simulink library "PczSimLib_R2020b"  (R2020b)
settings: Solver=VariableStepAuto  StartTime=0.0  StopTime=10.0  RelTol=1e-3
undefined symbols (not defined in the file or in its folder): beta, qc_get_step_size
libraries: dspswit3 x6, pid_lib x4, simulink x3
(part 1 of 2)
settings Model: Creator=SZTAKI  LastModifiedBy=SZTAKI

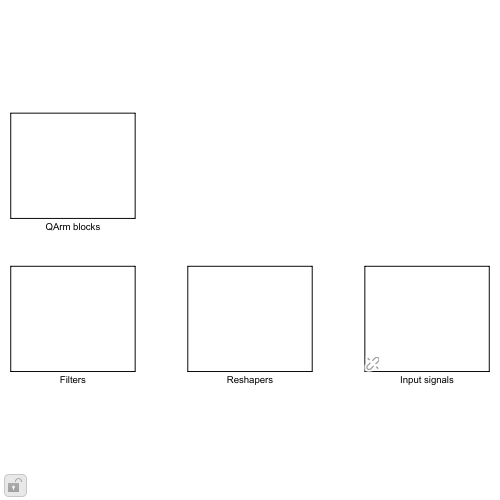
[thumbnail: Simulink's stored preview of the top-level diagram]
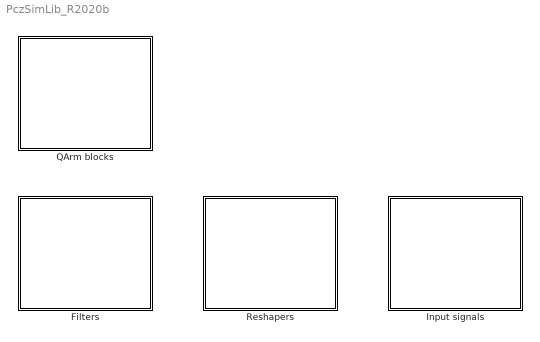
== system PczSimLib_R2020b ==
  Filters : Subsystem
  Input signals : Subsystem  AncestorBlock=PczSimLib_R2020b/Reshapers
  QArm blocks : Subsystem
  Reshapers : Subsystem

== system PczSimLib_R2020b/Filters ==
  Filter Tset = 0.05 [sec] : TransferFcn  Numerator=[0 0 0 1]  Denominator=[5.0000e-07 1.5000e-04 0.0200 1]
  Filter Tset = 0.1 [sec] : TransferFcn  Numerator=[0 0 0 1]  Denominator=[8.5000e-07 2.2000e-04 0.0270 1]
  Filter Tset = 0.25 [sec] : TransferFcn  Numerator=[0 0 0 1]  Denominator=[2.0000e-05 0.0022 0.0800 1]
  Filter Tset = 0.4 [sec] : TransferFcn  Numerator=[0 0 0 1]  Denominator=[7.0000e-05 0.0045 0.1200 1]
  Filter Tset = 0.7 [sec] : TransferFcn  Numerator=[0 0 0 0 0 1]  Denominator=[2.5000e-07 2.5000e-05 0.0011 0.0235 0.2500 1]
  Second-order low-pass filter : Subsystem

== system PczSimLib_R2020b/Input signals ==
  Sigmoid Steps : Subsystem

== system PczSimLib_R2020b/QArm blocks ==
  Current to pwm (corrected) 2022.04.28.1 : Subsystem
  Current transformed to pwm DEPRECATED : Subsystem
  PWM limiter I. : Subsystem
  PWM limiter II. : Subsystem
  Torque to pwm DEPRECATED : Subsystem
  Torque to pwm (J1-3 corrected) DEPRECATED : Subsystem
  Torque to pwm (corrected) 2022.04.28. : Subsystem
  Torque to pwm (corrected) velocity update 2022.05.20. : Subsystem
  "Torque to pwm (corrected) velocity update, current controlled 2022.05.20." : Subsystem
  XM430-W350-R characteristics (wrist) (corrected) : Subsystem
  "XM540-W270-R characteristics (base, shoulder, elbow) (corrected)" : Subsystem
  phi2theta : Subsystem
  theta2phi : Subsystem

== system PczSimLib_R2020b/Reshapers ==
  note: Reshaper = [4 3]; strjoin(cellfun(@(n) {num2str(n)},num2cell(reshape(reshape(1:prod(Reshaper),Reshaper)',[prod(Reshaper) 1])')),',')
  2x4 to 4x2 : Subsystem
  2x8 to 8x2 : Subsystem
  3x4 to 4x3 : Subsystem
  4x4 to 4x4 : Subsystem

== system PczSimLib_R2020b/Filters/Second-order low-pass filter ==
  x : Inport
  wn : Inport  Port=2
  zt : Inport  Port=3
  x0 : Inport  Port=4
  Constant : Constant  Value=2
  Integrator1 : Integrator  InitialConditionSource=external
  Integrator2 : Integrator
  Product : Product  RndMeth=Zero
  Product1 : Product  RndMeth=Zero
  Product2 : Product  Inputs=3  RndMeth=Zero
  Sum : Sum  Inputs=|+-
  Sum1 : Sum  Inputs=|+-
  y : Outport
  yd : Outport  Port=2
  wires:
  x0/1 -> Integrator1/2
  x/1 -> Sum1/1
  Integrator1/1 -> y/1, Sum1/2
  Constant/1 -> Product2/2
  Sum1/1 -> Sum/1
  Product2/1 -> Sum/2
  zt/1 -> Product2/3
  wn/1 -> Product1/1, Product/1
  Product1/1 -> yd/1, Integrator1/1
  Sum/1 -> Product/2
  Integrator2/1 -> Product2/1, Product1/2
  Product/1 -> Integrator2/1

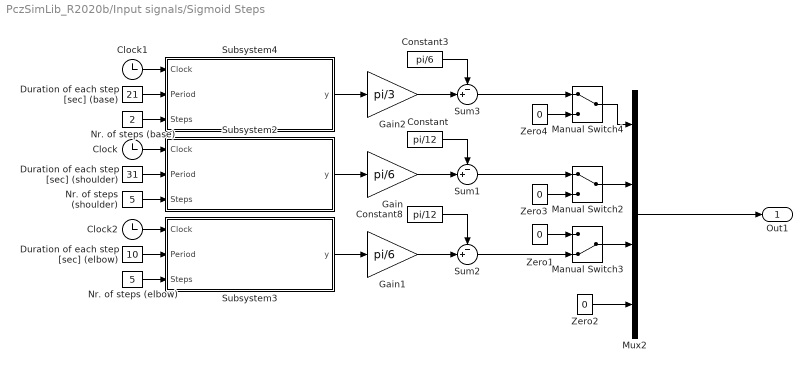
== system PczSimLib_R2020b/Input signals/Sigmoid Steps ==
  Clock : Clock
  Clock1 : Clock
  Clock2 : Clock
  Constant : Constant  Value=pi/12
  Constant3 : Constant  Value=pi/6
  Constant8 : Constant  Value=pi/12
  Duration of each step [sec] (base) : Constant  Value=21
  Duration of each step [sec] (elbow) : Constant  Value=10
  Duration of each step [sec] (shoulder) : Constant  Value=31
  Gain : Gain  Gain=pi/6
  Gain1 : Gain  Gain=pi/6
  Gain2 : Gain  Gain=pi/3
  Manual Switch2 : ManualSwitch
  Manual Switch3 : ManualSwitch  CurrentSetting=0
  Manual Switch4 : ManualSwitch
  Mux2 : Mux
  Nr. of steps (base) : Constant  Value=2
  Nr. of steps (elbow) : Constant  Value=5
  Nr. of steps (shoulder) : Constant  Value=5
  Subsystem2 : Subsystem
  Subsystem3 : Subsystem
  Subsystem4 : Subsystem
  Sum1 : Sum  Inputs=-+|
  Sum2 : Sum  Inputs=-+|
  Sum3 : Sum  Inputs=-+|
  Zero{1..4} (4 alike) : Constant  Value=0  OutDataTypeStr=Inherit: Inherit via back propagation
  Out1 : Outport
  wires:
  Manual Switch2/1 -> Mux2/2
  Duration of each step [sec] (shoulder)/1 -> Subsystem2/2(Period)
  Mux2/1 -> Out1/1
  Nr. of steps (base)/1 -> Subsystem4/3(Steps)
  Constant/1 -> Sum1/1
  Subsystem3/1(y) -> Gain1/1
  Nr. of steps (shoulder)/1 -> Subsystem2/3(Steps)
  Zero4/1 -> Manual Switch4/2
  Sum1/1 -> Manual Switch2/1
  Subsystem2/1(y) -> Gain/1
  Zero1/1 -> Manual Switch3/1
  Clock2/1 -> Subsystem3/1(Clock)
  Clock/1 -> Subsystem2/1(Clock)
  Zero3/1 -> Manual Switch2/2
  Constant3/1 -> Sum3/1
  Clock1/1 -> Subsystem4/1(Clock)
  Gain1/1 -> Sum2/2
  Duration of each step [sec] (elbow)/1 -> Subsystem3/2(Period)
  Subsystem4/1(y) -> Gain2/1
  Sum3/1 -> Manual Switch4/1
  Zero2/1 -> Mux2/4
  Manual Switch4/1 -> Mux2/1
  Constant8/1 -> Sum2/1
  Nr. of steps (elbow)/1 -> Subsystem3/3(Steps)
  Duration of each step [sec] (base)/1 -> Subsystem4/2(Period)
  Gain/1 -> Sum1/2
  Manual Switch3/1 -> Mux2/3
  Gain2/1 -> Sum3/2
  Sum2/1 -> Manual Switch3/2

== system PczSimLib_R2020b/QArm blocks/Current to pwm (corrected) 2022.04.28.1 ==
  current [4] : Inport
  angular vel [4] : Inport  Port=2
  M_curvel2pwm (2022.04.28.) : Constant  Value=|
      | [2.970000e-01,-1.400000e-03, 2.400000e-03,-9.800000e-03
      | -1.000000e-04, 8.800000e-02, 3.500000e-03,-0.000000e+00
      |  7.000000e-04, 8.400000e-03, 1.789000e-01,-2.600000e-03
      |  4.970000e-02, 2.830000e-02, 1.079000e-01, 6.711000e-01
      |  3.084000e-01, 4.800000e-03, 5.600000e-03, 1.100000e-03
      |  8.000000e-04, 3.198000e-01,-4.000000e-04, 5.500000e-03
      | -1.500000e-03,-1.110000e-02, 3.114000e-01, 7.800000e-03
      |  9.000000e-04,-2.300000e-03,-5.100000e-03, 2.074000e-01]'
  Mux2 : Mux  Inputs=2
  Product : Product  Multiplication=Matrix(*)
  pwm [4] : Outport
  wires:
  Mux2/1 -> Product/2
  M_curvel2pwm (2022.04.28.)/1 -> Product/1
  angular vel [4]/1 -> Mux2/2
  current [4]/1 -> Mux2/1
  Product/1 -> pwm [4]/1

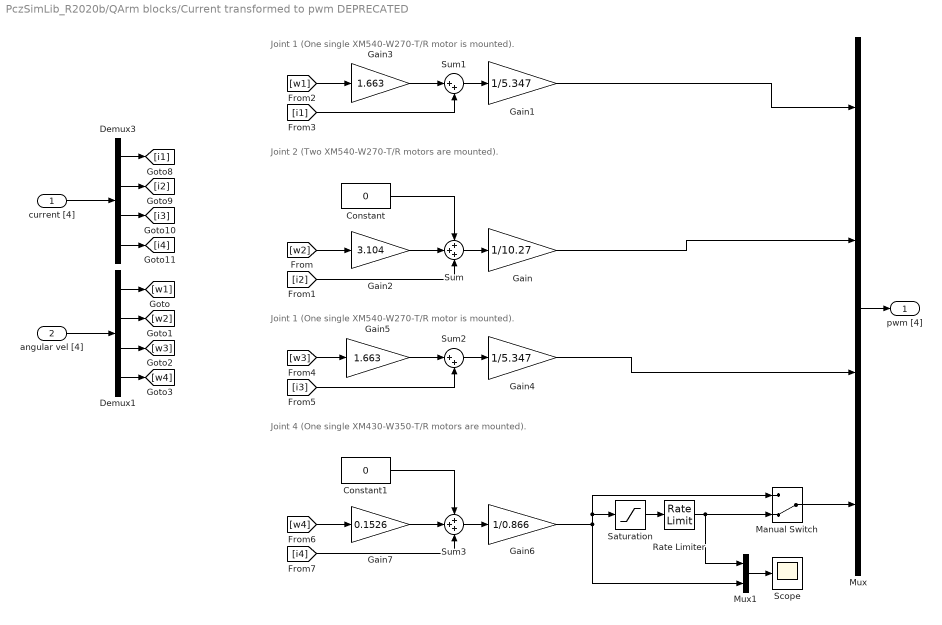
== system PczSimLib_R2020b/QArm blocks/Current transformed to pwm DEPRECATED ==
  note: Joint 4 (One single XM430-W350-T/R motors are mounted).
  note: Joint 1 (One single XM540-W270-T/R motor is mounted).
  note: Joint 1 (One single XM540-W270-T/R motor is mounted).
  note: Joint 2 (Two XM540-W270-T/R motors are mounted).
  current [4] : Inport
  angular vel [4] : Inport  Port=2
  Constant : Constant  Value=0
  Constant1 : Constant  Value=0
  Demux1 : Demux
  Demux3 : Demux
  Gain : Gain  Gain=1/10.27
  Gain1 : Gain  Gain=1/5.347
  Gain2 : Gain  Gain=3.104
  Gain3 : Gain  Gain=1.663
  Gain4 : Gain  Gain=1/5.347
  Gain5 : Gain  Gain=1.663
  Gain6 : Gain  Gain=1/0.866
  Gain7 : Gain  Gain=0.1526
  Manual Switch : ManualSwitch  CurrentSetting=0
  Mux : Mux
  Mux1 : Mux  Inputs=2
  Rate Limiter : RateLimiter  SampleTimeMode=inherited
  Saturation : Saturate  UpperLimit=0.4  LowerLimit=-0.4
  Scope : Scope
  Sum : Sum  Inputs=+++
  Sum1 : Sum  Inputs=|++
  Sum2 : Sum  Inputs=|++
  Sum3 : Sum  Inputs=+++
  pwm [4] : Outport
  wires:
  Manual Switch/1 -> Mux/4
  Mux1/1 -> Scope/1
  Rate Limiter/1 -> Mux1/1, Manual Switch/2
  Saturation/1 -> Rate Limiter/1
  Gain6/1 -> Mux1/2, Saturation/1, Manual Switch/1
  [w4] -> Gain7/1
  Constant1/1 -> Sum3/1
  Gain7/1 -> Sum3/2
  [i4] -> Sum3/3
  Sum3/1 -> Gain6/1
  Mux/1 -> pwm [4]/1
  Gain4/1 -> Mux/3
  Gain/1 -> Mux/2
  Gain1/1 -> Mux/1
  Sum2/1 -> Gain4/1
  [w3] -> Gain5/1
  Gain5/1 -> Sum2/1
  [i3] -> Sum2/2
  [i1] -> Sum1/2
  Gain3/1 -> Sum1/1
  [w1] -> Gain3/1
  Sum1/1 -> Gain1/1
  Sum/1 -> Gain/1
  [i2] -> Sum/3
  Gain2/1 -> Sum/2
  Constant/1 -> Sum/1
  [w2] -> Gain2/1
  current [4]/1 -> Demux3/1
  Demux3/4 -> [i4]
  Demux3/1 -> [i1]
  Demux3/2 -> [i2]
  Demux3/3 -> [i3]
  angular vel [4]/1 -> Demux1/1
  Demux1/1 -> [w1]
  Demux1/2 -> [w2]
  Demux1/3 -> [w3]
  Demux1/4 -> [w4]

== system PczSimLib_R2020b/QArm blocks/PWM limiter I. ==
  pwm in : Inport
  Demux : Demux
  Mux : Mux
  Rate Limiter{,1..3} (4 alike) : RateLimiter  RisingSlewLimit=2  FallingSlewLimit=-2  SampleTimeMode=inherited
  Saturation{,1..3} (4 alike) : Saturate  UpperLimit=0.8  LowerLimit=-0.8
  pwm out : Outport
  wires:
  Demux/4 -> Saturation2/1
  Demux/3 -> Saturation3/1
  Demux/2 -> Saturation1/1
  Demux/1 -> Saturation/1
  pwm in/1 -> Demux/1
  Saturation/1 -> Rate Limiter/1
  Saturation1/1 -> Rate Limiter1/1
  Saturation3/1 -> Rate Limiter2/1
  Saturation2/1 -> Rate Limiter3/1
  Rate Limiter3/1 -> Mux/4
  Rate Limiter2/1 -> Mux/3
  Rate Limiter1/1 -> Mux/2
  Rate Limiter/1 -> Mux/1
  Mux/1 -> pwm out/1

== system PczSimLib_R2020b/QArm blocks/PWM limiter II. ==
  pwm in : Inport
  Demux : Demux
  Mux : Mux
  Rate Limiter : RateLimiter  RisingSlewLimit=2  FallingSlewLimit=-2  SampleTimeMode=inherited
  Rate Limiter1 : RateLimiter  RisingSlewLimit=5  FallingSlewLimit=-5  SampleTimeMode=inherited
  Rate Limiter2 : RateLimiter  RisingSlewLimit=2  FallingSlewLimit=-2  SampleTimeMode=inherited
  Rate Limiter3 : RateLimiter  RisingSlewLimit=2  FallingSlewLimit=-2  SampleTimeMode=inherited
  Saturation{,1..3} (4 alike) : Saturate  UpperLimit=0.8  LowerLimit=-0.8
  pwm out : Outport
  wires:
  Mux/1 -> pwm out/1
  Rate Limiter/1 -> Mux/1
  Rate Limiter1/1 -> Mux/2
  Rate Limiter2/1 -> Mux/3
  Rate Limiter3/1 -> Mux/4
  Saturation2/1 -> Rate Limiter3/1
  Saturation3/1 -> Rate Limiter2/1
  Saturation1/1 -> Rate Limiter1/1
  Saturation/1 -> Rate Limiter/1
  pwm in/1 -> Demux/1
  Demux/1 -> Saturation/1
  Demux/2 -> Saturation1/1
  Demux/3 -> Saturation3/1
  Demux/4 -> Saturation2/1

== system PczSimLib_R2020b/QArm blocks/Torque to pwm DEPRECATED ==
  x [8] : Inport
  u [4] : Inport  Port=2
  params [17] : Inport  Port=3
  Constant1 : Constant  Value=0
  Mux1 : Mux  Inputs=2
  Selector : Selector  InputPortWidth=4  IndexOptions=Index vector (dialog)  Indices=1:3  OutputSizes=1
  Selector1 : Selector  InputPortWidth=8  IndexOptions=Index vector (dialog)  Indices=5:8  OutputSizes=1
  Selector2 : Selector  InputPortWidth=4  IndexOptions=Index vector (dialog)  Indices=4  OutputSizes=1
  Tau(u,x) : MATLAB Function  TreatAsAtomicUnit=on
  XM430-W350-R characteristics (corrected) : Subsystem
  XM540-W270-R characteristics (corrected) : Subsystem
  current transformed to pwm (corrected) : Subsystem
  pwm [4] : Outport
  i [4] : Outport  Port=2
  tau [4] : Outport  Port=3
  wires:
  current transformed to pwm (corrected)/1(pwm [4]) -> pwm [4]/1
  Mux1/1 -> i [4]/1, current transformed to pwm (corrected)/1(current [4])
  x [8]/1 -> Selector1/1, Tau(u,x)/3(x)
  Constant1/1 -> Tau(u,x)/4(mL)
  Selector/1 -> XM540-W270-R characteristics (corrected)/1(torque [3])
  XM540-W270-R characteristics (corrected)/1(current [3]) -> Mux1/1
  u [4]/1 -> Tau(u,x)/2(u)
  Tau(u,x)/1(Tau) -> tau [4]/1, Selector2/1, Selector/1  "Tau"
  Selector1/1 -> current transformed to pwm (corrected)/2(angular vel [4])
  Selector2/1 -> XM430-W350-R characteristics (corrected)/1(wrist torque)
  XM430-W350-R characteristics (corrected)/1(wrist current) -> Mux1/2
  params [17]/1 -> Tau(u,x)/1(params)

== system PczSimLib_R2020b/QArm blocks/Torque to pwm (J1-3 corrected) DEPRECATED ==
  x [8] : Inport
  u [4] : Inport  Port=2
  params [17] : Inport  Port=3
  Constant1 : Constant  Value=0
  Mux1 : Mux  Inputs=2
  Selector : Selector  InputPortWidth=4  IndexOptions=Index vector (dialog)  Indices=1:3  OutputSizes=1
  Selector1 : Selector  InputPortWidth=8  IndexOptions=Index vector (dialog)  Indices=5:8  OutputSizes=1
  Selector2 : Selector  InputPortWidth=4  IndexOptions=Index vector (dialog)  Indices=4  OutputSizes=1
  Tau(u,x) : MATLAB Function  TreatAsAtomicUnit=on
  XM430-W350-R characteristics (corrected) : Subsystem
  XM540-W270-R characteristics (corrected) : Subsystem
  current transformed to pwm (corrected) : Subsystem
  pwm [4] : Outport
  i [4] : Outport  Port=2
  tau [4] : Outport  Port=3
  wires:
  params [17]/1 -> Tau(u,x)/1(params)
  XM430-W350-R characteristics (corrected)/1(wrist current) -> Mux1/2
  Selector2/1 -> XM430-W350-R characteristics (corrected)/1(wrist torque)
  Selector1/1 -> current transformed to pwm (corrected)/2(angular vel [4])
  Tau(u,x)/1(Tau) -> Selector/1, Selector2/1, tau [4]/1  "Tau"
  u [4]/1 -> Tau(u,x)/2(u)
  XM540-W270-R characteristics (corrected)/1(current [3]) -> Mux1/1
  Selector/1 -> XM540-W270-R characteristics (corrected)/1(torque [3])
  Constant1/1 -> Tau(u,x)/4(mL)
  x [8]/1 -> Tau(u,x)/3(x), Selector1/1
  Mux1/1 -> current transformed to pwm (corrected)/1(current [4]), i [4]/1
  current transformed to pwm (corrected)/1(pwm [4]) -> pwm [4]/1

== system PczSimLib_R2020b/QArm blocks/Torque to pwm (corrected) 2022.04.28. ==
  x [8] : Inport
  u [4] : Inport  Port=2
  params [17] : Inport  Port=3
  Constant1 : Constant  Value=0
  Current to pwm (corrected) 2022.04.28. : Subsystem
  Mux1 : Mux  Inputs=2
  Selector : Selector  InputPortWidth=4  IndexOptions=Index vector (dialog)  Indices=1:3  OutputSizes=1
  Selector1 : Selector  InputPortWidth=8  IndexOptions=Index vector (dialog)  Indices=5:8  OutputSizes=1
  Selector2 : Selector  InputPortWidth=4  IndexOptions=Index vector (dialog)  Indices=4  OutputSizes=1
  Tau(u,x) : MATLAB Function  TreatAsAtomicUnit=on
  XM430-W350-R characteristics (corrected) : Subsystem
  XM540-W270-R characteristics (corrected) : Subsystem
  pwm [4] : Outport
  i [4] : Outport  Port=2
  tau [4] : Outport  Port=3
  wires:
  Current to pwm (corrected) 2022.04.28./1(pwm [4]) -> pwm [4]/1
  Mux1/1 -> Current to pwm (corrected) 2022.04.28./1(current [4]), i [4]/1
  x [8]/1 -> Selector1/1, Tau(u,x)/3(x)
  Constant1/1 -> Tau(u,x)/4(mL)
  Selector/1 -> XM540-W270-R characteristics (corrected)/1(torque [3])
  XM540-W270-R characteristics (corrected)/1(current [3]) -> Mux1/1
  u [4]/1 -> Tau(u,x)/2(u)
  Tau(u,x)/1(Tau) -> tau [4]/1, Selector2/1, Selector/1  "Tau"
  Selector1/1 -> Current to pwm (corrected) 2022.04.28./2(angular vel [4])
  Selector2/1 -> XM430-W350-R characteristics (corrected)/1(wrist torque)
  XM430-W350-R characteristics (corrected)/1(wrist current) -> Mux1/2
  params [17]/1 -> Tau(u,x)/1(params)

== system PczSimLib_R2020b/QArm blocks/Torque to pwm (corrected) velocity update 2022.05.20. ==
  x (Tc) [8] : Inport
  u (Tc) [4] : Inport  Port=2
  params [17] : Inport  Port=3
  w (Ts) [4] : Inport  Port=4
  Constant1 : Constant  Value=0
  Current to pwm (corrected) 2022.04.28. : Subsystem
  Mux1 : Mux  Inputs=2
  "Oversampling (Tc -> Ts)" : RateTransition  OutPortSampleTime=qc_get_step_size
  Selector : Selector  InputPortWidth=4  IndexOptions=Index vector (dialog)  Indices=1:3  OutputSizes=1
  Selector2 : Selector  InputPortWidth=4  IndexOptions=Index vector (dialog)  Indices=4  OutputSizes=1
  Tau(u,x) : MATLAB Function  TreatAsAtomicUnit=on
  XM430-W350-R characteristics (corrected) : Subsystem
  XM540-W270-R characteristics (corrected) : Subsystem
  pwm [4] : Outport
  i [4] : Outport  Port=2
  tau [4] : Outport  Port=3
  wires:
  params [17]/1 -> Tau(u,x)/1(params)
  XM430-W350-R characteristics (corrected)/1(wrist current) -> Mux1/2
  Selector2/1 -> XM430-W350-R characteristics (corrected)/1(wrist torque)
  Tau(u,x)/1(Tau) -> Selector/1, Selector2/1, tau [4]/1  "Tau"
  u (Tc) [4]/1 -> Tau(u,x)/2(u)
  XM540-W270-R characteristics (corrected)/1(current [3]) -> Mux1/1
  Selector/1 -> XM540-W270-R characteristics (corrected)/1(torque [3])
  Constant1/1 -> Tau(u,x)/4(mL)
  x (Tc) [8]/1 -> Tau(u,x)/3(x)
  Mux1/1 -> "Oversampling (Tc -> Ts)"/1, i [4]/1
  Current to pwm (corrected) 2022.04.28./1(pwm [4]) -> pwm [4]/1
  "Oversampling (Tc -> Ts)"/1 -> Current to pwm (corrected) 2022.04.28./1(current [4])
  w (Ts) [4]/1 -> Current to pwm (corrected) 2022.04.28./2(angular vel [4])

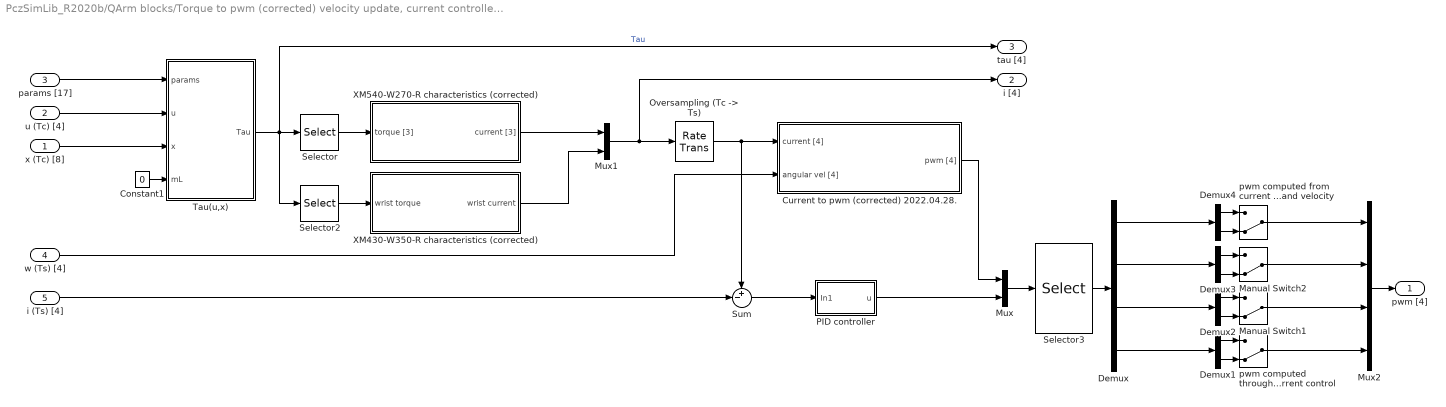
== system PczSimLib_R2020b/QArm blocks/Torque to pwm (corrected) velocity update, current controlled 2022.05.20. ==
  x (Tc) [8] : Inport
  u (Tc) [4] : Inport  Port=2
  params [17] : Inport  Port=3
  w (Ts) [4] : Inport  Port=4
  i (Ts) [4] : Inport  Port=5
  Constant1 : Constant  Value=0
  Current to pwm (corrected) 2022.04.28. : Subsystem
  Demux : Demux  Outputs=[2 2 2 2]
  Demux{1..4} (4 alike) : Demux  Outputs=2
  Manual Switch1 : ManualSwitch  CurrentSetting=0
  Manual Switch2 : ManualSwitch  CurrentSetting=0
  Mux : Mux  Inputs=2
  Mux1 : Mux  Inputs=2
  Mux2 : Mux
  "Oversampling (Tc -> Ts)" : RateTransition  OutPortSampleTime=qc_get_step_size
  PID controller : Subsystem
  Selector : Selector  InputPortWidth=4  IndexOptions=Index vector (dialog)  Indices=1:3  OutputSizes=1
  Selector2 : Selector  InputPortWidth=4  IndexOptions=Index vector (dialog)  Indices=4  OutputSizes=1
  Selector3 : Selector  InputPortWidth=8  IndexOptions=Index vector (dialog)  Indices=[1,5,2,6,3,7,4,8]  OutputSizes=1
  Sum : Sum  Inputs=+-|
  Tau(u,x) : MATLAB Function  TreatAsAtomicUnit=on
  XM430-W350-R characteristics (corrected) : Subsystem
  XM540-W270-R characteristics (corrected) : Subsystem
  pwm computed from current and velocity : ManualSwitch  CurrentSetting=0
  pwm computed through PID-based current control : ManualSwitch  CurrentSetting=0
  pwm [4] : Outport
  i [4] : Outport  Port=2
  tau [4] : Outport  Port=3
  wires:
  w (Ts) [4]/1 -> Current to pwm (corrected) 2022.04.28./2(angular vel [4])
  "Oversampling (Tc -> Ts)"/1 -> Current to pwm (corrected) 2022.04.28./1(current [4]), Sum/1
  Mux1/1 -> i [4]/1, "Oversampling (Tc -> Ts)"/1
  x (Tc) [8]/1 -> Tau(u,x)/3(x)
  Constant1/1 -> Tau(u,x)/4(mL)
  Selector/1 -> XM540-W270-R characteristics (corrected)/1(torque [3])
  XM540-W270-R characteristics (corrected)/1(current [3]) -> Mux1/1
  u (Tc) [4]/1 -> Tau(u,x)/2(u)
  Tau(u,x)/1(Tau) -> tau [4]/1, Selector2/1, Selector/1  "Tau"
  Selector2/1 -> XM430-W350-R characteristics (corrected)/1(wrist torque)
  XM430-W350-R characteristics (corrected)/1(wrist current) -> Mux1/2
  params [17]/1 -> Tau(u,x)/1(params)
  Manual Switch1/1 -> Mux2/3
  Manual Switch2/1 -> Mux2/2
  pwm computed through PID-based current control/1 -> Mux2/4
  Demux/4 -> Demux1/1
  Demux1/2 -> pwm computed through PID-based current control/2
  Demux/2 -> Demux3/1
  Current to pwm (corrected) 2022.04.28./1(pwm [4]) -> Mux/1
  PID controller/1(u) -> Mux/2
  Demux2/1 -> Manual Switch1/1
  Demux3/2 -> Manual Switch2/2
  Demux1/1 -> pwm computed through PID-based current control/1
  Demux3/1 -> Manual Switch2/1
  Demux2/2 -> Manual Switch1/2
  Demux/3 -> Demux2/1
  Selector3/1 -> Demux/1
  Mux/1 -> Selector3/1
  Demux/1 -> Demux4/1
  Demux4/1 -> pwm computed from current and velocity/1
  Demux4/2 -> pwm computed from current and velocity/2
  pwm computed from current and velocity/1 -> Mux2/1
  Mux2/1 -> pwm [4]/1
  Sum/1 -> PID controller/1(In1)
  i (Ts) [4]/1 -> Sum/2

== system PczSimLib_R2020b/QArm blocks/XM430-W350-R characteristics (wrist) (corrected) ==
  wrist torque : Inport
  Abs : Abs
  Constant : Constant  Value=0.0799
  Gain : Gain  Gain=1.7143
  Gain2 : Gain  Gain=0.5734
  Product : Product
  Sign : Signum
  Sum1 : Sum  Inputs=++|
  Switch : Switch  Criteria=u2 > Threshold  Threshold=0.07
  wrist current : Outport
  wires:
  Sign/1 -> Product/2
  Abs/1 -> Gain2/1, Gain/1, Switch/2
  Product/1 -> wrist current/1
  Constant/1 -> Sum1/1
  Gain2/1 -> Sum1/2
  wrist torque/1 -> Sign/1, Abs/1
  Gain/1 -> Switch/3
  Switch/1 -> Product/1  "wrist current"
  Sum1/1 -> Switch/1

== system PczSimLib_R2020b/QArm blocks/XM540-W270-R characteristics (base, shoulder, elbow) (corrected) ==
  torque [3] : Inport
  Abs : Abs
  Constant : Constant  Value=0.1461
  Gain : Gain  Gain=0.6788
  Gain1 : Gain  Gain=0.01717
  Gain2 : Gain  Gain=0.3067
  Product : Product
  Sign : Signum
  Square : Math  Operator=square  SaturateOnIntegerOverflow=on
  Sum1 : Sum  Inputs=+++
  Switch : Switch  Criteria=u2 > Threshold  Threshold=0.4
  current [3] : Outport
  wires:
  Product/1 -> current [3]/1
  Sign/1 -> Product/2
  torque [3]/1 -> Abs/1, Sign/1
  Sum1/1 -> Switch/1
  Switch/1 -> Product/1  "current [3]"
  Square/1 -> Gain1/1
  Gain/1 -> Switch/3
  Gain2/1 -> Sum1/3
  Gain1/1 -> Sum1/2
  Abs/1 -> Switch/2, Gain2/1, Square/1, Gain/1
  Constant/1 -> Sum1/1

== system PczSimLib_R2020b/QArm blocks/phi2theta ==
  phi : Inport
  Constant5 : Constant  Value=beta
  Constant6 : Constant  Value=pi/2
  Demux : Demux
  Mux3 : Mux
  Sum : Sum  Inputs=-++
  Sum1 : Sum  Inputs=-+|
  theta : Outport
  wires:
  Sum/1 -> Mux3/2  "theta2"
  Sum1/1 -> Mux3/3  "theta3"
  Demux/3 -> Sum1/2  "phi3"
  Constant5/1 -> Sum/3, Sum1/1
  Constant6/1 -> Sum/1
  Demux/2 -> Sum/2  "phi2"
  Demux/1 -> Mux3/1  "phi1 = theta1"
  Demux/4 -> Mux3/4  "phi4 = theta4"
  Mux3/1 -> theta/1
  phi/1 -> Demux/1

== system PczSimLib_R2020b/QArm blocks/theta2phi ==
  theta : Inport
  Constant5 : Constant  Value=beta
  Constant6 : Constant  Value=pi/2
  Demux : Demux
  Mux3 : Mux
  Sum : Sum  Inputs=++-
  Sum1 : Sum  Inputs=++|
  phi : Outport
  wires:
  theta/1 -> Demux/1
  Mux3/1 -> phi/1
  Demux/4 -> Mux3/4  "theta4 = phi4"
  Demux/1 -> Mux3/1  "theta1 = phi1"
  Demux/2 -> Sum/2  "theta2"
  Constant6/1 -> Sum/1
  Constant5/1 -> Sum1/1, Sum/3
  Demux/3 -> Sum1/2  "theta3"
  Sum1/1 -> Mux3/3  "phi3"
  Sum/1 -> Mux3/2  "phi2"

== system PczSimLib_R2020b/Reshapers/2x4 to 4x2 ==
  Input 1 [4] : Inport
  Input 2 [4] : Inport  Port=2
  Demux : Demux  Outputs=[2 2 2 2]
  Mux : Mux  Inputs=2
  Reshape block vector (2x4 to 4x2) : Selector  InputPortWidth=8  IndexOptions=Index vector (dialog)  Indices=[1,5,2,6,3,7,4,8]  OutputSizes=1
  Out1 : Outport
  Out2 : Outport  Port=2
  Out3 : Outport  Port=3
  Out4 : Outport  Port=4
  wires:
  Demux/4 -> Out4/1
  Demux/3 -> Out3/1
  Demux/2 -> Out2/1
  Demux/1 -> Out1/1
  Reshape block vector (2x4 to 4x2)/1 -> Demux/1
  Mux/1 -> Reshape block vector (2x4 to 4x2)/1
  Input 2 [4]/1 -> Mux/2
  Input 1 [4]/1 -> Mux/1

== system PczSimLib_R2020b/Reshapers/2x8 to 8x2 ==
  Input 1 [8] : Inport
  Input 2 [8] : Inport  Port=2
  Demux : Demux  Outputs=[2 2 2 2 2 2 2 2]
  Mux : Mux  Inputs=2
  Reshape block vector (2x8 to 8x2) : Selector  InputPortWidth=16  IndexOptions=Index vector (dialog)  Indices=[1,9,2,10,3,11,4,12,5,13,6,14,7,15,8,16]  OutputSizes=1
  Out1 : Outport
  Out2 : Outport  Port=2
  Out3 : Outport  Port=3
  Out4 : Outport  Port=4
  Out5 : Outport  Port=5
  Out6 : Outport  Port=6
  Out7 : Outport  Port=7
  Out8 : Outport  Port=8
  wires:
  Input 1 [8]/1 -> Mux/1
  Input 2 [8]/1 -> Mux/2
  Mux/1 -> Reshape block vector (2x8 to 8x2)/1
  Reshape block vector (2x8 to 8x2)/1 -> Demux/1
  Demux/1 -> Out1/1
  Demux/2 -> Out2/1
  Demux/3 -> Out3/1
  Demux/4 -> Out4/1
  Demux/5 -> Out5/1
  Demux/6 -> Out6/1
  Demux/7 -> Out7/1
  Demux/8 -> Out8/1

== system PczSimLib_R2020b/Reshapers/3x4 to 4x3 ==
  Input 1 [4] : Inport
  Input 2 [4] : Inport  Port=2
  Input 3 [4] : Inport  Port=3
  Demux : Demux  Outputs=[3 3 3 3]
  Mux : Mux  Inputs=3
  Transpose block vector (3x4 to 4x3) : Selector  InputPortWidth=12  IndexOptions=Index vector (dialog)  Indices=[1,5,9,2,6,10,3,7,11,4,8,12]  OutputSizes=1
  Out1 : Outport
  Out2 : Outport  Port=2
  Out3 : Outport  Port=3
  Out4 : Outport  Port=4
  wires:
  Input 1 [4]/1 -> Mux/1
  Input 2 [4]/1 -> Mux/2
  Mux/1 -> Transpose block vector (3x4 to 4x3)/1
  Transpose block vector (3x4 to 4x3)/1 -> Demux/1
  Demux/1 -> Out1/1
  Demux/2 -> Out2/1
  Demux/3 -> Out3/1
  Demux/4 -> Out4/1
  Input 3 [4]/1 -> Mux/3

== system PczSimLib_R2020b/Reshapers/4x4 to 4x4 ==
  Input 1 [4] : Inport
  Input 2 [4] : Inport  Port=2
  Input 3 [4] : Inport  Port=3
  Input 4 [4] : Inport  Port=4
  Demux : Demux  Outputs=[4 4 4 4]
  Mux : Mux
  Transpose block vector (4x4 to 4x4) : Selector  InputPortWidth=16  IndexOptions=Index vector (dialog)  Indices=[1,5,9,13,2,6,10,14,3,7,11,15,4,8,12,16]  OutputSizes=1
  Out1 : Outport
  Out2 : Outport  Port=2
  Out3 : Outport  Port=3
  Out4 : Outport  Port=4
  wires:
  Input 4 [4]/1 -> Mux/4
  Input 3 [4]/1 -> Mux/3
  Demux/4 -> Out4/1
  Demux/3 -> Out3/1
  Demux/2 -> Out2/1
  Demux/1 -> Out1/1
  Transpose block vector (4x4 to 4x4)/1 -> Demux/1
  Mux/1 -> Transpose block vector (4x4 to 4x4)/1
  Input 2 [4]/1 -> Mux/2
  Input 1 [4]/1 -> Mux/1

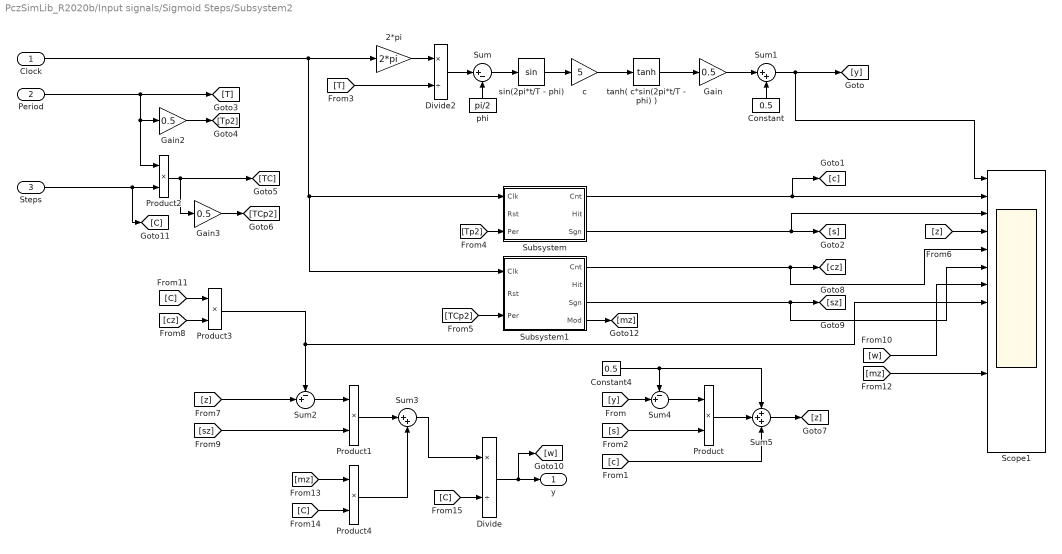
== system PczSimLib_R2020b/Input signals/Sigmoid Steps/Subsystem2 ==
  Clock : Inport
  Period : Inport  Port=2
  Steps : Inport  Port=3
  2*pi : Gain  Gain=2*pi
  Constant : Constant  Value=0.5
  Constant4 : Constant  Value=0.5
  Divide : Product  Inputs=*/
  Divide2 : Product  Inputs=*/
  Gain : Gain  Gain=0.5
  Gain2 : Gain  Gain=0.5
  Gain3 : Gain  Gain=0.5
  Product{,1..4} (5 alike) : Product
  Scope1 : Scope  NumInputPorts=16
  Subsystem : Subsystem
  Subsystem1 : Subsystem
  Sum : Sum  Inputs=|+-
  Sum1 : Sum  Inputs=|++
  Sum2 : Sum  Inputs=-+|
  Sum3 : Sum  Inputs=|++
  Sum4 : Sum  Inputs=-+|
  Sum5 : Sum  Inputs=+++
  c : Gain  Gain=5
  phi : Constant  Value=pi/2  OutDataTypeStr=Inherit: Inherit via back propagation
  sin(2pi*t/T - phi) : Trigonometry
  tanh( c*sin(2pi*t/T - phi) ) : Trigonometry  Operator=tanh
  y : Outport
  wires:
  [mz] -> Scope1/12
  Sum5/1 -> [z]
  [y] -> Sum4/2
  [C] -> Product3/1
  c/1 -> tanh( c*sin(2pi*t/T - phi) )/1
  Constant/1 -> Sum1/2
  Sum3/1 -> Divide/1
  [cz] -> Product3/2
  [z] -> Sum2/2
  Subsystem/3(Sgn) -> Scope1/3, [s]
  [s] -> Product/2
  Product1/1 -> Sum3/1
  Clock/1 -> Subsystem1/1(Clk), Subsystem/1(Clk), 2*pi/1
  Subsystem1/3(Sgn) -> Scope1/6, [sz]
  Sum2/1 -> Product1/1
  Product3/1 -> Sum2/1, Scope1/8
  Constant4/1 -> Sum5/1, Sum4/1
  Gain3/1 -> [TCp2]
  [z] -> Scope1/4
  sin(2pi*t/T - phi)/1 -> c/1
  2*pi/1 -> Divide2/1
  [T] -> Divide2/2
  [sz] -> Product1/2
  [c] -> Sum5/3
  [TCp2] -> Subsystem1/3(Per)
  Period/1 -> Product2/1, Gain2/1, [T]
  [mz] -> Product4/1
  Product4/1 -> Sum3/2
  Gain/1 -> Sum1/1
  phi/1 -> Sum/2
  Product/1 -> Sum5/2
  Subsystem1/1(Cnt) -> Scope1/5, [cz]
  Divide2/1 -> Sum/1
  [C] -> Product4/2
  tanh( c*sin(2pi*t/T - phi) )/1 -> Gain/1
  [Tp2] -> Subsystem/3(Per)
  Sum/1 -> sin(2pi*t/T - phi)/1
  Sum1/1 -> Scope1/1, [y]
  Gain2/1 -> [Tp2]
  Sum4/1 -> Product/1
  Steps/1 -> [C], Product2/2
  Subsystem1/4(Mod) -> [mz]
  [w] -> Scope1/7
  Product2/1 -> Gain3/1, [TC]
  Subsystem/1(Cnt) -> [c], Scope1/2
  Divide/1 -> y/1, [w]
  [C] -> Divide/2

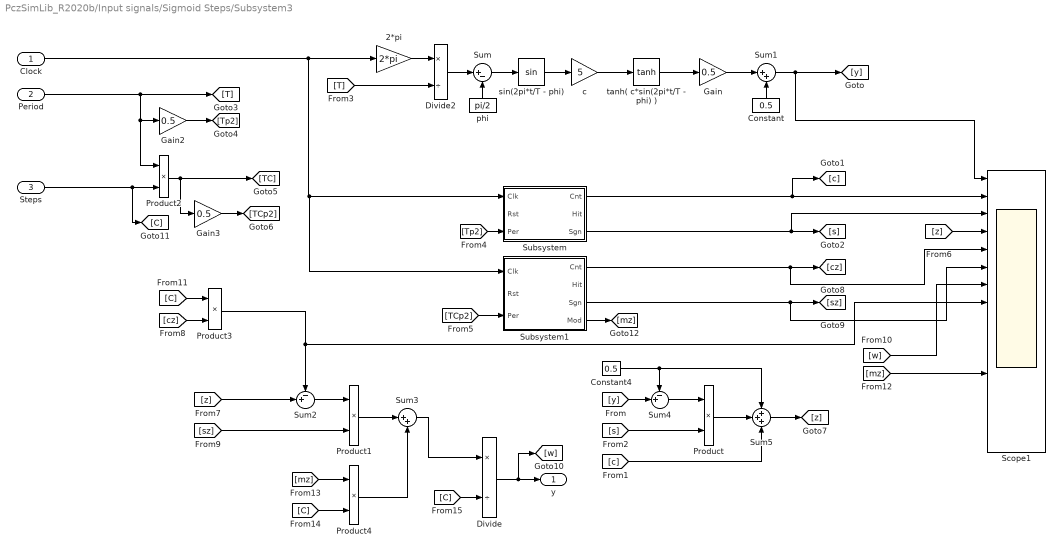
== system PczSimLib_R2020b/Input signals/Sigmoid Steps/Subsystem3 ==
  Clock : Inport
  Period : Inport  Port=2
  Steps : Inport  Port=3
  2*pi : Gain  Gain=2*pi
  Constant : Constant  Value=0.5
  Constant4 : Constant  Value=0.5
  Divide : Product  Inputs=*/
  Divide2 : Product  Inputs=*/
  Gain : Gain  Gain=0.5
  Gain2 : Gain  Gain=0.5
  Gain3 : Gain  Gain=0.5
  Product{,1..4} (5 alike) : Product
  Scope1 : Scope  NumInputPorts=16
  Subsystem : Subsystem
  Subsystem1 : Subsystem
  Sum : Sum  Inputs=|+-
  Sum1 : Sum  Inputs=|++
  Sum2 : Sum  Inputs=-+|
  Sum3 : Sum  Inputs=|++
  Sum4 : Sum  Inputs=-+|
  Sum5 : Sum  Inputs=+++
  c : Gain  Gain=5
  phi : Constant  Value=pi/2  OutDataTypeStr=Inherit: Inherit via back propagation
  sin(2pi*t/T - phi) : Trigonometry
  tanh( c*sin(2pi*t/T - phi) ) : Trigonometry  Operator=tanh
  y : Outport
  wires:
  [C] -> Divide/2
  Divide/1 -> [w], y/1
  Subsystem/1(Cnt) -> Scope1/2, [c]
  Product2/1 -> [TC], Gain3/1
  [w] -> Scope1/7
  Subsystem1/4(Mod) -> [mz]
  Steps/1 -> Product2/2, [C]
  Sum4/1 -> Product/1
  Gain2/1 -> [Tp2]
  Sum1/1 -> [y], Scope1/1
  Sum/1 -> sin(2pi*t/T - phi)/1
  [Tp2] -> Subsystem/3(Per)
  tanh( c*sin(2pi*t/T - phi) )/1 -> Gain/1
  [C] -> Product4/2
  Divide2/1 -> Sum/1
  Subsystem1/1(Cnt) -> [cz], Scope1/5
  Product/1 -> Sum5/2
  phi/1 -> Sum/2
  Gain/1 -> Sum1/1
  Product4/1 -> Sum3/2
  [mz] -> Product4/1
  Period/1 -> [T], Gain2/1, Product2/1
  [TCp2] -> Subsystem1/3(Per)
  [c] -> Sum5/3
  [sz] -> Product1/2
  [T] -> Divide2/2
  2*pi/1 -> Divide2/1
  sin(2pi*t/T - phi)/1 -> c/1
  [z] -> Scope1/4
  Gain3/1 -> [TCp2]
  Constant4/1 -> Sum4/1, Sum5/1
  Product3/1 -> Scope1/8, Sum2/1
  Sum2/1 -> Product1/1
  Subsystem1/3(Sgn) -> [sz], Scope1/6
  Clock/1 -> 2*pi/1, Subsystem/1(Clk), Subsystem1/1(Clk)
  Product1/1 -> Sum3/1
  [s] -> Product/2
  Subsystem/3(Sgn) -> [s], Scope1/3
  [z] -> Sum2/2
  [cz] -> Product3/2
  Sum3/1 -> Divide/1
  Constant/1 -> Sum1/2
  c/1 -> tanh( c*sin(2pi*t/T - phi) )/1
  [C] -> Product3/1
  [y] -> Sum4/2
  Sum5/1 -> [z]
  [mz] -> Scope1/12

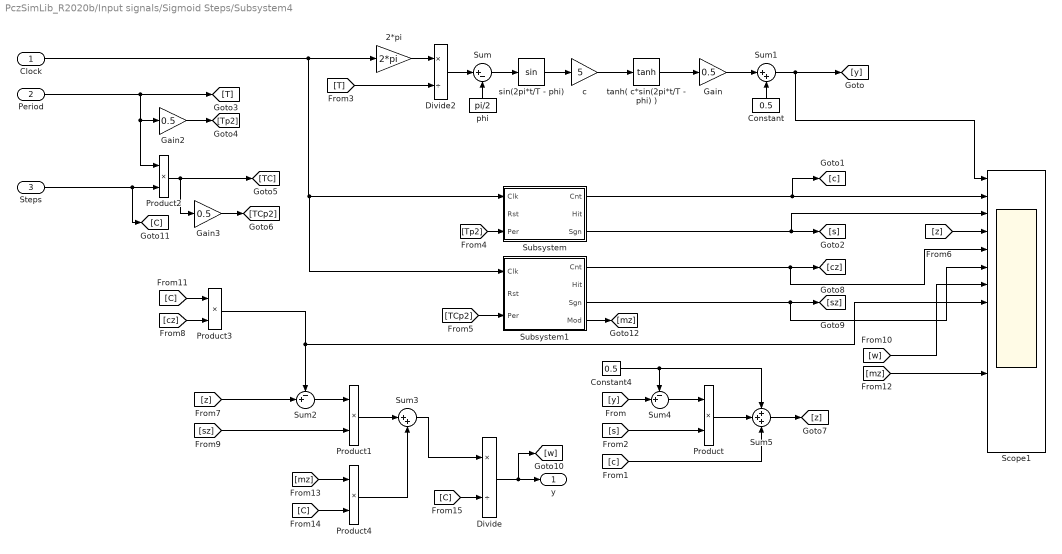
== system PczSimLib_R2020b/Input signals/Sigmoid Steps/Subsystem4 ==
  Clock : Inport
  Period : Inport  Port=2
  Steps : Inport  Port=3
  2*pi : Gain  Gain=2*pi
  Constant : Constant  Value=0.5
  Constant4 : Constant  Value=0.5
  Divide : Product  Inputs=*/
  Divide2 : Product  Inputs=*/
  Gain : Gain  Gain=0.5
  Gain2 : Gain  Gain=0.5
  Gain3 : Gain  Gain=0.5
  Product{,1..4} (5 alike) : Product
  Scope1 : Scope  NumInputPorts=16
  Subsystem : Subsystem
  Subsystem1 : Subsystem
  Sum : Sum  Inputs=|+-
  Sum1 : Sum  Inputs=|++
  Sum2 : Sum  Inputs=-+|
  Sum3 : Sum  Inputs=|++
  Sum4 : Sum  Inputs=-+|
  Sum5 : Sum  Inputs=+++
  c : Gain  Gain=5
  phi : Constant  Value=pi/2  OutDataTypeStr=Inherit: Inherit via back propagation
  sin(2pi*t/T - phi) : Trigonometry
  tanh( c*sin(2pi*t/T - phi) ) : Trigonometry  Operator=tanh
  y : Outport
  wires:
  [C] -> Divide/2
  Divide/1 -> [w], y/1
  Subsystem/1(Cnt) -> Scope1/2, [c]
  Product2/1 -> [TC], Gain3/1
  [w] -> Scope1/7
  Subsystem1/4(Mod) -> [mz]
  Steps/1 -> Product2/2, [C]
  Sum4/1 -> Product/1
  Gain2/1 -> [Tp2]
  Sum1/1 -> [y], Scope1/1
  Sum/1 -> sin(2pi*t/T - phi)/1
  [Tp2] -> Subsystem/3(Per)
  tanh( c*sin(2pi*t/T - phi) )/1 -> Gain/1
  [C] -> Product4/2
  Divide2/1 -> Sum/1
  Subsystem1/1(Cnt) -> [cz], Scope1/5
  Product/1 -> Sum5/2
  phi/1 -> Sum/2
  Gain/1 -> Sum1/1
  Product4/1 -> Sum3/2
  [mz] -> Product4/1
  Period/1 -> [T], Gain2/1, Product2/1
  [TCp2] -> Subsystem1/3(Per)
  [c] -> Sum5/3
  [sz] -> Product1/2
  [T] -> Divide2/2
  2*pi/1 -> Divide2/1
  sin(2pi*t/T - phi)/1 -> c/1
  [z] -> Scope1/4
  Gain3/1 -> [TCp2]
  Constant4/1 -> Sum4/1, Sum5/1
  Product3/1 -> Scope1/8, Sum2/1
  Sum2/1 -> Product1/1
  Subsystem1/3(Sgn) -> [sz], Scope1/6
  Clock/1 -> 2*pi/1, Subsystem/1(Clk), Subsystem1/1(Clk)
  Product1/1 -> Sum3/1
  [s] -> Product/2
  Subsystem/3(Sgn) -> [s], Scope1/3
  [z] -> Sum2/2
  [cz] -> Product3/2
  Sum3/1 -> Divide/1
  Constant/1 -> Sum1/2
  c/1 -> tanh( c*sin(2pi*t/T - phi) )/1
  [C] -> Product3/1
  [y] -> Sum4/2
  Sum5/1 -> [z]
  [mz] -> Scope1/12

== system PczSimLib_R2020b/QArm blocks/Torque to pwm DEPRECATED/XM430-W350-R characteristics (corrected) ==
  wrist torque : Inport
  Abs : Abs
  Constant : Constant  Value=0.0799
  Gain : Gain  Gain=1.7143
  Gain2 : Gain  Gain=0.5734
  Product : Product
  Sign : Signum
  Sum1 : Sum  Inputs=++|
  Switch : Switch  Criteria=u2 > Threshold  Threshold=0.07
  wrist current : Outport
  wires:
  Sum1/1 -> Switch/1
  Switch/1 -> Product/1  "wrist current"
  Gain/1 -> Switch/3
  wrist torque/1 -> Abs/1, Sign/1
  Gain2/1 -> Sum1/2
  Constant/1 -> Sum1/1
  Product/1 -> wrist current/1
  Abs/1 -> Switch/2, Gain/1, Gain2/1
  Sign/1 -> Product/2

== system PczSimLib_R2020b/QArm blocks/Torque to pwm DEPRECATED/XM540-W270-R characteristics (corrected) ==
  torque [3] : Inport
  Abs : Abs
  Constant : Constant  Value=0.1461
  Gain : Gain  Gain=0.6788
  Gain1 : Gain  Gain=0.01717
  Gain2 : Gain  Gain=0.3067
  Product : Product
  Sign : Signum
  Square : Math  Operator=square  SaturateOnIntegerOverflow=on
  Sum1 : Sum  Inputs=+++
  Switch : Switch  Criteria=u2 > Threshold  Threshold=0.4
  current [3] : Outport
  wires:
  Constant/1 -> Sum1/1
  Abs/1 -> Gain/1, Square/1, Gain2/1, Switch/2
  Gain1/1 -> Sum1/2
  Gain2/1 -> Sum1/3
  Gain/1 -> Switch/3
  Square/1 -> Gain1/1
  Switch/1 -> Product/1  "current [3]"
  Sum1/1 -> Switch/1
  torque [3]/1 -> Sign/1, Abs/1
  Sign/1 -> Product/2
  Product/1 -> current [3]/1

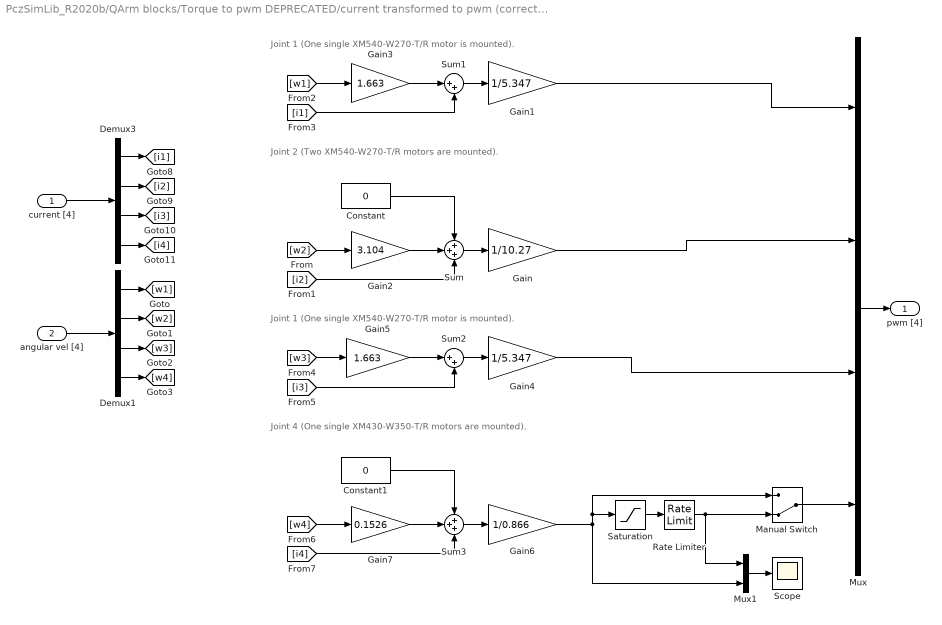
== system PczSimLib_R2020b/QArm blocks/Torque to pwm DEPRECATED/current transformed to pwm (corrected) ==
  note: Joint 2 (Two XM540-W270-T/R motors are mounted).
  note: Joint 1 (One single XM540-W270-T/R motor is mounted).
  note: Joint 1 (One single XM540-W270-T/R motor is mounted).
  note: Joint 4 (One single XM430-W350-T/R motors are mounted).
  current [4] : Inport
  angular vel [4] : Inport  Port=2
  Constant : Constant  Value=0
  Constant1 : Constant  Value=0
  Demux1 : Demux
  Demux3 : Demux
  Gain : Gain  Gain=1/10.27
  Gain1 : Gain  Gain=1/5.347
  Gain2 : Gain  Gain=3.104
  Gain3 : Gain  Gain=1.663
  Gain4 : Gain  Gain=1/5.347
  Gain5 : Gain  Gain=1.663
  Gain6 : Gain  Gain=1/0.866
  Gain7 : Gain  Gain=0.1526
  Manual Switch : ManualSwitch  CurrentSetting=0
  Mux : Mux
  Mux1 : Mux  Inputs=2
  Rate Limiter : RateLimiter  SampleTimeMode=inherited
  Saturation : Saturate  UpperLimit=0.4  LowerLimit=-0.4
  Scope : Scope
  Sum : Sum  Inputs=+++
  Sum1 : Sum  Inputs=|++
  Sum2 : Sum  Inputs=|++
  Sum3 : Sum  Inputs=+++
  pwm [4] : Outport
  wires:
  Demux1/4 -> [w4]
  Demux1/3 -> [w3]
  Demux1/2 -> [w2]
  Demux1/1 -> [w1]
  angular vel [4]/1 -> Demux1/1
  Demux3/3 -> [i3]
  Demux3/2 -> [i2]
  Demux3/1 -> [i1]
  Demux3/4 -> [i4]
  current [4]/1 -> Demux3/1
  [w2] -> Gain2/1
  Constant/1 -> Sum/1
  Gain2/1 -> Sum/2
  [i2] -> Sum/3
  Sum/1 -> Gain/1
  Sum1/1 -> Gain1/1
  [w1] -> Gain3/1
  Gain3/1 -> Sum1/1
  [i1] -> Sum1/2
  [i3] -> Sum2/2
  Gain5/1 -> Sum2/1
  [w3] -> Gain5/1
  Sum2/1 -> Gain4/1
  Gain1/1 -> Mux/1
  Gain/1 -> Mux/2
  Gain4/1 -> Mux/3
  Mux/1 -> pwm [4]/1
  Sum3/1 -> Gain6/1
  [i4] -> Sum3/3
  Gain7/1 -> Sum3/2
  Constant1/1 -> Sum3/1
  [w4] -> Gain7/1
  Gain6/1 -> Manual Switch/1, Saturation/1, Mux1/2
  Saturation/1 -> Rate Limiter/1
  Rate Limiter/1 -> Manual Switch/2, Mux1/1
  Mux1/1 -> Scope/1
  Manual Switch/1 -> Mux/4

== system PczSimLib_R2020b/QArm blocks/Torque to pwm (J1-3 corrected) DEPRECATED/XM430-W350-R characteristics (corrected) ==
  wrist torque : Inport
  Abs : Abs
  Constant : Constant  Value=0.0799
  Gain : Gain  Gain=1.7143
  Gain2 : Gain  Gain=0.5734
  Product : Product
  Sign : Signum
  Sum1 : Sum  Inputs=++|
  Switch : Switch  Criteria=u2 > Threshold  Threshold=0.07
  wrist current : Outport
  wires:
  Sign/1 -> Product/2
  Abs/1 -> Gain2/1, Gain/1, Switch/2
  Product/1 -> wrist current/1
  Constant/1 -> Sum1/1
  Gain2/1 -> Sum1/2
  wrist torque/1 -> Sign/1, Abs/1
  Gain/1 -> Switch/3
  Switch/1 -> Product/1  "wrist current"
  Sum1/1 -> Switch/1

== system PczSimLib_R2020b/QArm blocks/Torque to pwm (J1-3 corrected) DEPRECATED/XM540-W270-R characteristics (corrected) ==
  torque [3] : Inport
  Abs : Abs
  Constant : Constant  Value=0.1461
  Gain : Gain  Gain=0.6788
  Gain1 : Gain  Gain=0.01717
  Gain2 : Gain  Gain=0.3067
  Product : Product
  Sign : Signum
  Square : Math  Operator=square  SaturateOnIntegerOverflow=on
  Sum1 : Sum  Inputs=+++
  Switch : Switch  Criteria=u2 > Threshold  Threshold=0.4
  current [3] : Outport
  wires:
  Product/1 -> current [3]/1
  Sign/1 -> Product/2
  torque [3]/1 -> Abs/1, Sign/1
  Sum1/1 -> Switch/1
  Switch/1 -> Product/1  "current [3]"
  Square/1 -> Gain1/1
  Gain/1 -> Switch/3
  Gain2/1 -> Sum1/3
  Gain1/1 -> Sum1/2
  Abs/1 -> Switch/2, Gain2/1, Square/1, Gain/1
  Constant/1 -> Sum1/1

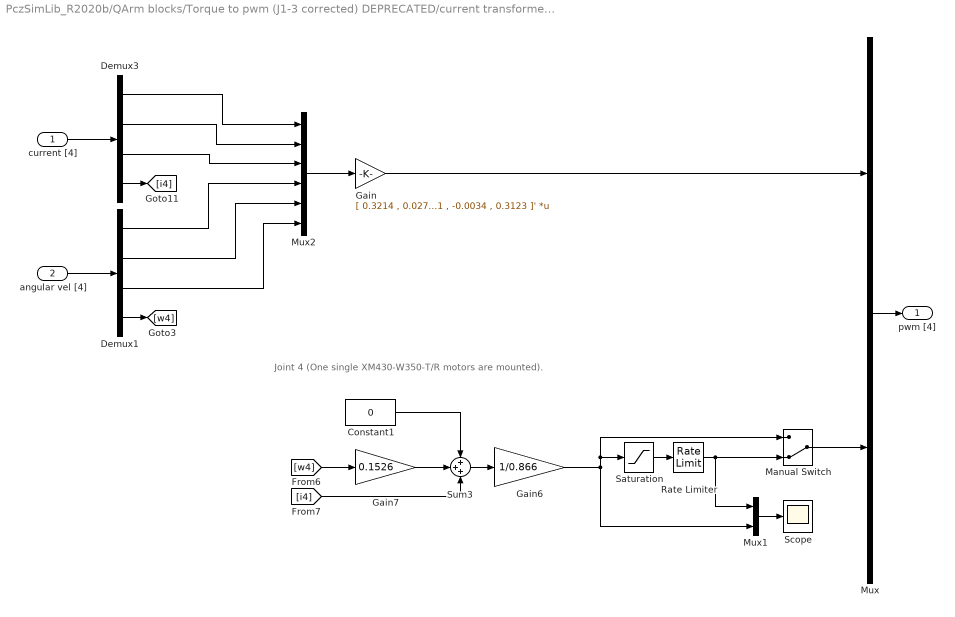
== system PczSimLib_R2020b/QArm blocks/Torque to pwm (J1-3 corrected) DEPRECATED/current transformed to pwm (corrected) ==
  note: Joint 4 (One single XM430-W350-T/R motors are mounted).
  current [4] : Inport
  angular vel [4] : Inport  Port=2
  Constant1 : Constant  Value=0
  Demux1 : Demux
  Demux3 : Demux
  Gain : Gain  Gain=[ 0.3214 , 0.0277 , 0.0036 ; 0.0001 , 0.0943 , 0.0026 ; -0.0002 , 0.0046 , 0.1848 ; 0.2811 , 0.0024 , 0.0023 ; -0.0002 , 0.3018 , -0.009 ; 0.001 , -0.0034 , 0.3123 ]'  Multiplication=Matrix(K*u) (u vector)
  Gain6 : Gain  Gain=1/0.866
  Gain7 : Gain  Gain=0.1526
  Manual Switch : ManualSwitch  CurrentSetting=0
  Mux : Mux  Inputs=2
  Mux1 : Mux  Inputs=2
  Mux2 : Mux  Inputs=6
  Rate Limiter : RateLimiter  SampleTimeMode=inherited
  Saturation : Saturate  UpperLimit=0.4  LowerLimit=-0.4
  Scope : Scope
  Sum3 : Sum  Inputs=+++
  pwm [4] : Outport
  wires:
  Manual Switch/1 -> Mux/2
  Mux1/1 -> Scope/1
  Rate Limiter/1 -> Mux1/1, Manual Switch/2
  Saturation/1 -> Rate Limiter/1
  Gain6/1 -> Mux1/2, Saturation/1, Manual Switch/1
  [w4] -> Gain7/1
  Constant1/1 -> Sum3/1
  Gain7/1 -> Sum3/2
  [i4] -> Sum3/3
  Sum3/1 -> Gain6/1
  Mux/1 -> pwm [4]/1
  current [4]/1 -> Demux3/1
  Demux3/4 -> [i4]
  angular vel [4]/1 -> Demux1/1
  Demux1/4 -> [w4]
  Demux3/1 -> Mux2/1
  Demux3/2 -> Mux2/2
  Demux3/3 -> Mux2/3
  Demux1/1 -> Mux2/4
  Demux1/2 -> Mux2/5
  Demux1/3 -> Mux2/6
  Mux2/1 -> Gain/1
  Gain/1 -> Mux/1

== system PczSimLib_R2020b/QArm blocks/Torque to pwm (corrected) 2022.04.28./Current to pwm (corrected) 2022.04.28. ==
  current [4] : Inport
  angular vel [4] : Inport  Port=2
  M_curvel2pwm (2022.04.28.) : Constant  Value=|
      | [2.970000e-01,-1.400000e-03, 2.400000e-03,-9.800000e-03
      | -1.000000e-04, 8.800000e-02, 3.500000e-03,-0.000000e+00
      |  7.000000e-04, 8.400000e-03, 1.789000e-01,-2.600000e-03
      |  4.970000e-02, 2.830000e-02, 1.079000e-01, 6.711000e-01
      |  3.084000e-01, 4.800000e-03, 5.600000e-03, 1.100000e-03
      |  8.000000e-04, 3.198000e-01,-4.000000e-04, 5.500000e-03
      | -1.500000e-03,-1.110000e-02, 3.114000e-01, 7.800000e-03
      |  9.000000e-04,-2.300000e-03,-5.100000e-03, 2.074000e-01]'
  Mux2 : Mux  Inputs=2
  Product : Product  Multiplication=Matrix(*)
  pwm [4] : Outport
  wires:
  Product/1 -> pwm [4]/1
  current [4]/1 -> Mux2/1
  angular vel [4]/1 -> Mux2/2
  M_curvel2pwm (2022.04.28.)/1 -> Product/1
  Mux2/1 -> Product/2

== system PczSimLib_R2020b/QArm blocks/Torque to pwm (corrected) 2022.04.28./XM430-W350-R characteristics (corrected) ==
  wrist torque : Inport
  Abs : Abs
  Constant : Constant  Value=0.0799
  Gain : Gain  Gain=1.7143
  Gain2 : Gain  Gain=0.5734
  Product : Product
  Sign : Signum
  Sum1 : Sum  Inputs=++|
  Switch : Switch  Criteria=u2 > Threshold  Threshold=0.07
  wrist current : Outport
  wires:
  Sum1/1 -> Switch/1
  Switch/1 -> Product/1  "wrist current"
  Gain/1 -> Switch/3
  wrist torque/1 -> Abs/1, Sign/1
  Gain2/1 -> Sum1/2
  Constant/1 -> Sum1/1
  Product/1 -> wrist current/1
  Abs/1 -> Switch/2, Gain/1, Gain2/1
  Sign/1 -> Product/2

== system PczSimLib_R2020b/QArm blocks/Torque to pwm (corrected) 2022.04.28./XM540-W270-R characteristics (corrected) ==
  torque [3] : Inport
  Abs : Abs
  Constant : Constant  Value=0.1461
  Gain : Gain  Gain=0.6788
  Gain1 : Gain  Gain=0.01717
  Gain2 : Gain  Gain=0.3067
  Product : Product
  Sign : Signum
  Square : Math  Operator=square  SaturateOnIntegerOverflow=on
  Sum1 : Sum  Inputs=+++
  Switch : Switch  Criteria=u2 > Threshold  Threshold=0.4
  current [3] : Outport
  wires:
  Constant/1 -> Sum1/1
  Abs/1 -> Gain/1, Square/1, Gain2/1, Switch/2
  Gain1/1 -> Sum1/2
  Gain2/1 -> Sum1/3
  Gain/1 -> Switch/3
  Square/1 -> Gain1/1
  Switch/1 -> Product/1  "current [3]"
  Sum1/1 -> Switch/1
  torque [3]/1 -> Sign/1, Abs/1
  Sign/1 -> Product/2
  Product/1 -> current [3]/1

== system PczSimLib_R2020b/QArm blocks/Torque to pwm (corrected) velocity update 2022.05.20./Current to pwm (corrected) 2022.04.28. ==
  current [4] : Inport
  angular vel [4] : Inport  Port=2
  M_curvel2pwm (2022.04.28.) : Constant  Value=|
      | [2.970000e-01,-1.400000e-03, 2.400000e-03,-9.800000e-03
      | -1.000000e-04, 8.800000e-02, 3.500000e-03,-0.000000e+00
      |  7.000000e-04, 8.400000e-03, 1.789000e-01,-2.600000e-03
      |  4.970000e-02, 2.830000e-02, 1.079000e-01, 6.711000e-01
      |  3.084000e-01, 4.800000e-03, 5.600000e-03, 1.100000e-03
      |  8.000000e-04, 3.198000e-01,-4.000000e-04, 5.500000e-03
      | -1.500000e-03,-1.110000e-02, 3.114000e-01, 7.800000e-03
      |  9.000000e-04,-2.300000e-03,-5.100000e-03, 2.074000e-01]'
  Mux2 : Mux  Inputs=2
  Product : Product  Multiplication=Matrix(*)
  pwm [4] : Outport
  wires:
  Mux2/1 -> Product/2
  M_curvel2pwm (2022.04.28.)/1 -> Product/1
  angular vel [4]/1 -> Mux2/2
  current [4]/1 -> Mux2/1
  Product/1 -> pwm [4]/1

== system PczSimLib_R2020b/QArm blocks/Torque to pwm (corrected) velocity update 2022.05.20./XM430-W350-R characteristics (corrected) ==
  wrist torque : Inport
  Abs : Abs
  Constant : Constant  Value=0.0799
  Gain : Gain  Gain=1.7143
  Gain2 : Gain  Gain=0.5734
  Product : Product
  Sign : Signum
  Sum1 : Sum  Inputs=++|
  Switch : Switch  Criteria=u2 > Threshold  Threshold=0.07
  wrist current : Outport
  wires:
  Sign/1 -> Product/2
  Abs/1 -> Gain2/1, Gain/1, Switch/2
  Product/1 -> wrist current/1
  Constant/1 -> Sum1/1
  Gain2/1 -> Sum1/2
  wrist torque/1 -> Sign/1, Abs/1
  Gain/1 -> Switch/3
  Switch/1 -> Product/1  "wrist current"
  Sum1/1 -> Switch/1

== system PczSimLib_R2020b/QArm blocks/Torque to pwm (corrected) velocity update 2022.05.20./XM540-W270-R characteristics (corrected) ==
  torque [3] : Inport
  Abs : Abs
  Constant : Constant  Value=0.1461
  Gain : Gain  Gain=0.6788
  Gain1 : Gain  Gain=0.01717
  Gain2 : Gain  Gain=0.3067
  Product : Product
  Sign : Signum
  Square : Math  Operator=square  SaturateOnIntegerOverflow=on
  Sum1 : Sum  Inputs=+++
  Switch : Switch  Criteria=u2 > Threshold  Threshold=0.4
  current [3] : Outport
  wires:
  Product/1 -> current [3]/1
  Sign/1 -> Product/2
  torque [3]/1 -> Abs/1, Sign/1
  Sum1/1 -> Switch/1
  Switch/1 -> Product/1  "current [3]"
  Square/1 -> Gain1/1
  Gain/1 -> Switch/3
  Gain2/1 -> Sum1/3
  Gain1/1 -> Sum1/2
  Abs/1 -> Switch/2, Gain2/1, Square/1, Gain/1
  Constant/1 -> Sum1/1

== system PczSimLib_R2020b/QArm blocks/Torque to pwm (corrected) velocity update, current controlled 2022.05.20./Current to pwm (corrected) 2022.04.28. ==
  current [4] : Inport
  angular vel [4] : Inport  Port=2
  M_curvel2pwm (2022.04.28.) : Constant  Value=|
      | [2.970000e-01,-1.400000e-03, 2.400000e-03,-9.800000e-03
      | -1.000000e-04, 8.800000e-02, 3.500000e-03,-0.000000e+00
      |  7.000000e-04, 8.400000e-03, 1.789000e-01,-2.600000e-03
      |  4.970000e-02, 2.830000e-02, 1.079000e-01, 6.711000e-01
      |  3.084000e-01, 4.800000e-03, 5.600000e-03, 1.100000e-03
      |  8.000000e-04, 3.198000e-01,-4.000000e-04, 5.500000e-03
      | -1.500000e-03,-1.110000e-02, 3.114000e-01, 7.800000e-03
      |  9.000000e-04,-2.300000e-03,-5.100000e-03, 2.074000e-01]'
  Mux2 : Mux  Inputs=2
  Product : Product  Multiplication=Matrix(*)
  pwm [4] : Outport
  wires:
  Product/1 -> pwm [4]/1
  current [4]/1 -> Mux2/1
  angular vel [4]/1 -> Mux2/2
  M_curvel2pwm (2022.04.28.)/1 -> Product/1
  Mux2/1 -> Product/2

== system PczSimLib_R2020b/QArm blocks/Torque to pwm (corrected) velocity update, current controlled 2022.05.20./PID controller ==
  In1 : Inport
  Demux : Demux
  Mux : Mux
  PID Controller{,1..3} (4 alike) : pid_lib/PID Controller  Controller=PID  Form=Parallel  TimeDomain=Discrete-time  UseExternalTs=off  SampleTime=qc_get_step_size  IntegratorMethod=Forward Euler  FilterMethod=Forward Euler  ControllerParametersSource=internal  P=0.635  I=2.58  D=-0.0585  UseFilter=on  N=1/0.0935  TunerSelectOption=Transfer Function Based (PID Tuner App)  InitialConditionSource=internal  InitialConditionForIntegrator=0  InitialConditionForFilter=0  DifferentiatorICPrevScaledInput=0  ExternalReset=none  TrackingMode=off  Kt=1  LimitOutput=on  SatLimitsSource=internal  UpperSaturationLimit=0.8  LowerSaturationLimit=-0.8  LinearizeAsGain=on  AntiWindupMode=back-calculation  Kb=0.5  POutMin=[]  POutMax=[]  IOutMin=[]  IOutMax=[]  DOutMin=[]  DOutMax=[]  NOutMin=[]  NOutMax=[]  SumOutMin=[]  SumOutMax=[]  SaturationOutMin=[]  SaturationOutMax=[]  PParamMin=[]  PParamMax=[]  IParamMin=[]  IParamMax=[]  DParamMin=[]  DParamMax=[]  NParamMin=[]  NParamMax=[]  KbParamMin=[]  KbParamMax=[]  KtParamMin=[]  KtParamMax=[]  KbOutMin=[]  KbOutMax=[]  KtOutMin=[]  KtOutMax=[]  IntegratorOutMin=[]  IntegratorOutMax=[]  FilterOutMin=[]  FilterOutMax=[]  SumI1OutMin=[]  SumI1OutMax=[]  SumI2OutMin=[]  SumI2OutMax=[]  SumI3OutMin=[]  SumI3OutMax=[]  SumI4OutMin=[]  SumI4OutMax=[]  SumDOutMin=[]  SumDOutMax=[]  DifferentiatorOutMin=[]  DifferentiatorOutMax=[]  FilterDiffOutCoefMin=[]  FilterDiffOutCoefMax=[]  ReciprocalOutMin=[]  ReciprocalOutMax=[]  SumDenOutMin=[]  SumDenOutMax=[]  SumNumOutMin=[]  SumNumOutMax=[]  DivideOutMin=[]  DivideOutMax=[]  UdiffTsProdOutMin=[]  UdiffTsProdOutMax=[]  NTsProdOutMin=[]  NTsProdOutMax=[]  UintegralTsProdOutMin=[]  UintegralTsProdOutMax=[]  UngainTsProdOutMin=[]  UngainTsProdOutMax=[]  IntegratorContinuousStateAttributes=''  IntegratorStateMustResolveToSignalObject=off  IntegratorRTWStateStorageClass=Auto  FilterContinuousStateAttributes=''  FilterStateMustResolveToSignalObject=off  FilterRTWStateStorageClass=Auto  ParallelPVariant=InternalParameters  IdealPVariant=Disabled  IVariant=InternalParameters  DVariant=InternalParameters  IntegratorVariant=Discrete  SatVariant=Enabled  AWVariant=BackCalculation  PCopyVariant=Disabled  TRVariant=Disabled  FdbkBlocksVariant=Forward  IdealPFdbkVariant=Disabled  SatFdbkVariant=Disabled  DerivativeFilterVariant=ForwardEulerFilter  NVariant=InternalParameters  NCopyVariant=Disabled  FilterICVariant=InternalICsFilter  IntegratorICVariant=InternalICs  ExternalResetVariant=Disabled  TRSumVariant=Passthrough  SumFdbkVariant=Disabled  SumVariant=Sum_PID  TsampFilterVariant=InternalTs  TsampNgainVariant=Passthrough  TsampIntegralVariant=Passthrough  ExternalSaturationOutDataTypeStr=Inherit: Same as second input
  u : Outport
  wires:
  In1/1 -> Demux/1
  Demux/1 -> PID Controller2/1
  Mux/1 -> u/1
  PID Controller2/1 -> Mux/1
  PID Controller1/1 -> Mux/2
  PID Controller/1 -> Mux/3
  Demux/3 -> PID Controller/1
  Demux/2 -> PID Controller1/1
  Demux/4 -> PID Controller3/1
  PID Controller3/1 -> Mux/4

== system PczSimLib_R2020b/QArm blocks/Torque to pwm (corrected) velocity update, current controlled 2022.05.20./XM430-W350-R characteristics (corrected) ==
  wrist torque : Inport
  Abs : Abs
  Constant : Constant  Value=0.0799
  Gain : Gain  Gain=1.7143
  Gain2 : Gain  Gain=0.5734
  Product : Product
  Sign : Signum
  Sum1 : Sum  Inputs=++|
  Switch : Switch  Criteria=u2 > Threshold  Threshold=0.07
  wrist current : Outport
  wires:
  Sum1/1 -> Switch/1
  Switch/1 -> Product/1  "wrist current"
  Gain/1 -> Switch/3
  wrist torque/1 -> Abs/1, Sign/1
  Gain2/1 -> Sum1/2
  Constant/1 -> Sum1/1
  Product/1 -> wrist current/1
  Abs/1 -> Switch/2, Gain/1, Gain2/1
  Sign/1 -> Product/2

== system PczSimLib_R2020b/QArm blocks/Torque to pwm (corrected) velocity update, current controlled 2022.05.20./XM540-W270-R characteristics (corrected) ==
  torque [3] : Inport
  Abs : Abs
  Constant : Constant  Value=0.1461
  Gain : Gain  Gain=0.6788
  Gain1 : Gain  Gain=0.01717
  Gain2 : Gain  Gain=0.3067
  Product : Product
  Sign : Signum
  Square : Math  Operator=square  SaturateOnIntegerOverflow=on
  Sum1 : Sum  Inputs=+++
  Switch : Switch  Criteria=u2 > Threshold  Threshold=0.4
  current [3] : Outport
  wires:
  Constant/1 -> Sum1/1
  Abs/1 -> Gain/1, Square/1, Gain2/1, Switch/2
  Gain1/1 -> Sum1/2
  Gain2/1 -> Sum1/3
  Gain/1 -> Switch/3
  Square/1 -> Gain1/1
  Switch/1 -> Product/1  "current [3]"
  Sum1/1 -> Switch/1
  torque [3]/1 -> Sign/1, Abs/1
  Sign/1 -> Product/2
  Product/1 -> current [3]/1

== system PczSimLib_R2020b/Input signals/Sigmoid Steps/Subsystem2/Subsystem ==
  Clk : Inport
  Rst : Inport  Port=2
  Per : Inport  Port=3
  Constant1 : Constant
  Constant2 : Constant  Value=2
  Constant3 : Constant
  Counter : dspswit3/Counter  Direction=Up  CountEvent=Rising edge  CounterSize=User defined  MaxCount=255  InitialCount=0  Output=Count and Hit  HitValue=32  ResetInput=on  SamplesPerFrame=1  Ts=1  CntDtype=double  HitDtype=Logical
  Gain1 : Gain  Gain=-2
  GreaterThan : RelationalOperator  Operator=<  OutDataTypeStr=boolean  RndMeth=Simplest
  Memory : Memory
  Mod : Math  Operator=mod  SaturateOnIntegerOverflow=on
  Product1 : Product
  Sum2 : Sum  Inputs=++|
  Sum3 : Sum  Inputs=|++
  Cnt : Outport
  Hit : Outport  Port=2
  Sgn : Outport  Port=3
  wires:
  Counter/2 -> Hit/1
  Clk/1 -> GreaterThan/2
  Rst/1 -> Counter/2
  Memory/1 -> Sum2/2
  Constant3/1 -> Sum3/2
  Per/1 -> Product1/1
  GreaterThan/1 -> Counter/1
  Constant1/1 -> Sum2/1
  Sum2/1 -> Product1/2
  Constant2/1 -> Mod/2
  Gain1/1 -> Sum3/1
  Counter/1 -> Memory/1, Cnt/1, Mod/1  "Counter"
  Product1/1 -> GreaterThan/1
  Mod/1 -> Gain1/1
  Sum3/1 -> Sgn/1

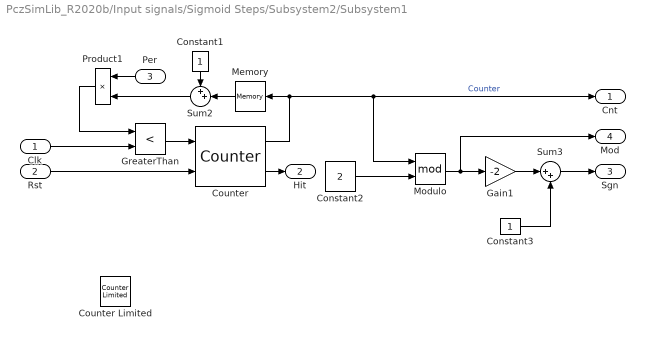
== system PczSimLib_R2020b/Input signals/Sigmoid Steps/Subsystem2/Subsystem1 ==
  Clk : Inport
  Rst : Inport  Port=2
  Per : Inport  Port=3
  Constant1 : Constant
  Constant2 : Constant  Value=2
  Constant3 : Constant
  Counter : dspswit3/Counter  Direction=Up  CountEvent=Rising edge  CounterSize=User defined  MaxCount=255  InitialCount=0  Output=Count and Hit  HitValue=32  ResetInput=on  SamplesPerFrame=1  Ts=1  CntDtype=double  HitDtype=Logical
  Counter Limited : simulink/Sources/Counter Limited  uplimit=7  tsamp=-1
  Gain1 : Gain  Gain=-2
  GreaterThan : RelationalOperator  Operator=<  OutDataTypeStr=boolean  RndMeth=Simplest
  Memory : Memory
  Modulo : Math  Operator=mod  SaturateOnIntegerOverflow=on
  Product1 : Product
  Sum2 : Sum  Inputs=++|
  Sum3 : Sum  Inputs=|++
  Cnt : Outport
  Hit : Outport  Port=2
  Sgn : Outport  Port=3
  Mod : Outport  Port=4
  wires:
  Sum3/1 -> Sgn/1
  Modulo/1 -> Mod/1, Gain1/1
  Product1/1 -> GreaterThan/1
  Counter/1 -> Modulo/1, Cnt/1, Memory/1  "Counter"
  Gain1/1 -> Sum3/1
  Constant2/1 -> Modulo/2
  Sum2/1 -> Product1/2
  Constant1/1 -> Sum2/1
  GreaterThan/1 -> Counter/1
  Per/1 -> Product1/1
  Constant3/1 -> Sum3/2
  Memory/1 -> Sum2/2
  Rst/1 -> Counter/2
  Clk/1 -> GreaterThan/2
  Counter/2 -> Hit/1
